simulink model "IdmEstimation_Cogen"  (R2017b)
settings: Solver=FixedStepDiscrete  StartTime=0.0  StopTime=SimTime  FixedStep=0.01  RelTol=1e-3
values from neighbouring files (symbols this model uses):
  BaseMap_CoastAccdiff_Index = (0:0.5:3.5)'    [IdmDev_MdlClassification.m]    (also in IdmParam.mat = [0 0.5 1 1.5 2 2.5 3 3.5]; IdmParam_Integ.mat = [0 0.5 1 1.5 2 2.5 3 3.5])
  BaseMap_CoastSpeed_Index = (5:5:40)'    [IdmDev_MdlClassification.m]    (also in IdmParam.mat = [5 10 15 20 25 30 35 40]; IdmParam_Integ.mat = [5 10 15 20 25 30 35 40])
  LrnConfig =     [ModelConfig.mat]
  ModelConfig =     [ModelConfig.mat]
  OnlineConfig =     [ModelConfig.mat]
  ParamCase = Fcn_ParamSelect(Param,Index_case)    [IdmDev_LearnSILsValidation.m]    (also in IdmDev_LearningOnlineSimulation.m)
undefined symbols (not defined in the file or in its folder): acc_veh, dis_veh, vel_veh
libraries: simulink x7
(part 2 of 2)

== system IdmEstimation_Cogen/IdmLrn_ParameterUpdate/Parameter update/MaxAccUpdate ==
  MaxAccRef : Inport
  MaxAcc : Inport  Port=2
  LrnFac : Inport  Port=3
  In4 : Inport  Port=4
  Constant1 : Constant  Value=LrnConfig.ExpUpdateGain
  Constant2 : Constant  Value=LrnConfig.LrnSwt
  Data Store Read : DataStoreRead  DataStoreName=IdmLrn_EcpParamVec_MaxAcc
  Data Store Write1 : DataStoreWrite  DataStoreName=IdmLrn_EcpParamVec_MaxAcc
  Divide : Product  Inputs=*/
  Product : Product
  Sum : Sum  Inputs=|+-
  Sum1 : Sum  Inputs=|++
  Switch : Switch  Criteria=u2 > Threshold  Threshold=0.5
  To Workspace : ToWorkspace  VariableName=LrnResult_EcpParamVec_MaxAcc  SaveFormat=Structure With Time  SampleTime=-1
  wires:
  Product/1 -> Divide/1  "TargetDelta"
  Sum/1 -> Product/1
  MaxAcc/1 -> Sum/2
  Switch/1 -> Product/2
  MaxAccRef/1 -> Sum/1
  LrnFac/1 -> Divide/2
  Divide/1 -> Sum1/1  "LrnValueVec"
  Data Store Read/1 -> Sum1/2
  Sum1/1 -> To Workspace/1, Data Store Write1/1
  Constant2/1 -> Switch/2
  In4/1 -> Switch/3
  Constant1/1 -> Switch/1

== system IdmEstimation_Cogen/IdmLrn_ParameterUpdate/Parameter update/TpDeltaUpdate ==
  TpStallRef : Inport
  TpStall : Inport  Port=2
  LrnFac : Inport  Port=3
  In4 : Inport  Port=4
  Constant : Constant  Value=LrnConfig.ExpUpdateGain
  Constant1 : Constant  Value=LrnConfig.LrnSwt
  Data Store Read2 : DataStoreRead  DataStoreName=IdmLrn_EcpParamVec_TpDelta
  Data Store Write3 : DataStoreWrite  DataStoreName=IdmLrn_EcpParamVec_TpDelta
  Divide : Product  Inputs=*/
  Product : Product
  Sum : Sum  Inputs=|+-
  Sum1 : Sum  Inputs=|++
  Switch : Switch  Criteria=u2 > Threshold  Threshold=0.5
  To Workspace : ToWorkspace  VariableName=LrnResult_EcpParamVec_TpDelta  SaveFormat=Structure With Time  SampleTime=-1
  wires:
  Sum1/1 -> To Workspace/1, Data Store Write3/1
  Data Store Read2/1 -> Sum1/2
  Divide/1 -> Sum1/1  "LrnValueVec"
  LrnFac/1 -> Divide/2
  TpStallRef/1 -> Sum/1
  Switch/1 -> Product/2
  TpStall/1 -> Sum/2
  Sum/1 -> Product/1
  Product/1 -> Divide/1  "TargetDelta"
  Constant1/1 -> Switch/2
  In4/1 -> Switch/3
  Constant/1 -> Switch/1

== system IdmEstimation_Cogen/IdmLrn_ParameterUpdate/Parameter update/TpInitUpdate ==
  TpInitRef : Inport
  TpInit : Inport  Port=2
  LrnFac : Inport  Port=3
  In4 : Inport  Port=4
  Constant : Constant  Value=LrnConfig.ExpUpdateGain
  Constant1 : Constant  Value=LrnConfig.LrnSwt
  Data Store Read2 : DataStoreRead  DataStoreName=IdmLrn_EcpParamVec_TpInit
  Data Store Write2 : DataStoreWrite  DataStoreName=IdmLrn_EcpParamVec_TpInit
  Display : Display
  Divide : Product  Inputs=*/
  Product : Product
  Sum : Sum  Inputs=|+-
  Sum1 : Sum  Inputs=|++
  Switch : Switch  Criteria=u2 > Threshold  Threshold=0.5
  To Workspace : ToWorkspace  VariableName=LrnResult_EcpParamVec_TpInit  SaveFormat=Structure With Time  SampleTime=-1
  wires:
  Product/1 -> Divide/1  "TargetDelta"
  Sum/1 -> Display/1, Product/1
  TpInit/1 -> Sum/2
  Constant/1 -> Switch/1
  TpInitRef/1 -> Sum/1
  LrnFac/1 -> Divide/2
  Divide/1 -> Sum1/1  "LrnValueVec"
  Data Store Read2/1 -> Sum1/2
  Sum1/1 -> To Workspace/1, Data Store Write2/1
  Constant1/1 -> Switch/2
  In4/1 -> Switch/3
  Switch/1 -> Product/2

== system IdmEstimation_Cogen/IdmEst_AccEstimation/Model profile update/Model profile update - Coast state/DisAdjCalc ==
  Constant : Constant  Value=0
  Mod_DisAdj : Outport
  wires:
  Constant/1 -> Mod_DisAdj/1

== system IdmEstimation_Cogen/IdmEst_AccEstimation/Model profile update/Model profile update - Coast state/DisDelCalc ==
  Constant : Constant  Value=0
  Mod_DisDel : Outport
  wires:
  Constant/1 -> Mod_DisDel/1

== system IdmEstimation_Cogen/IdmEst_AccEstimation/Model profile update/Model profile update - Coast state/RefAccCalc ==
  note: tmpLoc_ModProf_acc_ref(index_curstep+1) = -0.5*tmpLoc_Mod_vel_est(index_curstep+1).^2/(tmpLoc_Mod_dis_est(index_curstep+1) - DrvConfig.StopDis);
  Mod_VelEstPri : Inport
  Mod_DisEstPri : Inport  Port=2
  Constant : Constant  Value=ModelConfig.StopDis
  Constant1 : Constant  Value=-0.5
  Product : Product
  Product1 : Product  Inputs=**/
  Sum : Sum  Inputs=|+-
  Mod_AccRef : Outport
  wires:
  Mod_VelEstPri/1 -> Product/2, Product/1
  Product/1 -> Product1/2
  Constant1/1 -> Product1/1
  Mod_DisEstPri/1 -> Sum/1
  Constant/1 -> Sum/2
  Sum/1 -> Product1/3
  Product1/1 -> Mod_AccRef/1

== system IdmEstimation_Cogen/IdmEst_AccEstimation/Model profile update/Model profile update - Coast state/RefVelCalc ==
  Mod_VelRefPri : Inport
  AccEst : Inport  Port=2
  Constant : Constant  Value=OnlineConfig.Ts
  Product : Product
  Sum : Sum  Inputs=|++
  Mod_VelRef : Outport
  wires:
  Mod_VelRefPri/1 -> Sum/1
  Product/1 -> Sum/2
  Sum/1 -> Mod_VelRef/1
  Constant/1 -> Product/2
  AccEst/1 -> Product/1

== system IdmEstimation_Cogen/IdmEst_AccEstimation/Model profile update/Model profile update - Disadj state/DisAdjCalc ==
  Mod_DisEstPri : Inport
  Mod_DisAdj : Outport
  wires:
  Mod_DisEstPri/1 -> Mod_DisAdj/1

== system IdmEstimation_Cogen/IdmEst_AccEstimation/Model profile update/Model profile update - Disadj state/DisDelCalc ==
  Mod_DisDelPri : Inport
  ModelParam : Inport  Port=2
  In3 : Inport  Port=3
  Product : Product
  Selector : Selector  InputPortWidth=OnlineConfig.CalcParamSize  IndexOptions=Index vector (dialog)  Indices=OnlineConfig.CalcParamIndex.AccdDisAdj  OutputSizes=1
  Sum : Sum  Inputs=|++
  Mod_DisDel : Outport
  wires:
  Sum/1 -> Mod_DisDel/1
  ModelParam/1 -> Selector/1
  Selector/1 -> Product/1  "ModelParam_AccDiff"
  Mod_DisDelPri/1 -> Sum/1
  In3/1 -> Product/2
  Product/1 -> Sum/2

== system IdmEstimation_Cogen/IdmEst_AccEstimation/Model profile update/Model profile update - Disadj state/RefAccCalc ==
  note: tmpLoc_ModProf_acc_ref(index_curstep+1) = -0.5*tmpLoc_Mod_vel_est(index_curstep+1).^2/(tmpLoc_Mod_dis_est(index_curstep+1) - DrvConfig.StopDis);
  Mod_VelEstPri : Inport
  Mod_DisEstPri : Inport  Port=2
  Constant : Constant  Value=ModelConfig.StopDis
  Constant1 : Constant  Value=-0.5
  Product : Product
  Product1 : Product  Inputs=**/
  Sum : Sum  Inputs=|+-
  Mod_AccRef : Outport
  wires:
  Mod_VelEstPri/1 -> Product/2, Product/1
  Product/1 -> Product1/2
  Constant1/1 -> Product1/1
  Mod_DisEstPri/1 -> Sum/1
  Constant/1 -> Sum/2
  Sum/1 -> Product1/3
  Product1/1 -> Mod_AccRef/1

== system IdmEstimation_Cogen/IdmEst_AccEstimation/Model profile update/Model profile update - Disadj state/RefVelCalc ==
  Mod_VelEstPri : Inport
  Mod_DisEstPri : Inport  Port=2
  Mod_DisAdjPri : Inport  Port=3
  ModParam : Inport  Port=4
  Constant1 : Constant  Value=1/ModelConfig.Delta
  Math Function : Math  Operator=pow  SaturateOnIntegerOverflow=on
  Math Function1 : Math  Operator=square  SaturateOnIntegerOverflow=on
  Product : Product  Inputs=*/
  Product1 : Product  Inputs=*/
  Saturation : Saturate  UpperLimit=inf  LowerLimit=0.00001
  Selector : Selector  InputPortWidth=OnlineConfig.CalcParamSize  IndexOptions=Index vector (dialog)  Indices=OnlineConfig.CalcParamIndex.AccrStall  OutputSizes=1
  Sum1 : Sum  Inputs=|+-
  Mod_VelRef : Outport
  wires:
  Product/1 -> Mod_VelRef/1
  Mod_VelEstPri/1 -> Product/1
  ModParam/1 -> Selector/1
  Selector/1 -> Sum1/1  "ModParam_AccRatioFacStall"
  Mod_DisAdjPri/1 -> Product1/1
  Mod_DisEstPri/1 -> Product1/2
  Sum1/1 -> Saturation/1
  Constant1/1 -> Math Function/2
  Math Function/1 -> Product/2
  Product1/1 -> Math Function1/1
  Math Function1/1 -> Sum1/2
  Saturation/1 -> Math Function/1

== system IdmEstimation_Cogen/IdmEst_AccEstimation/Model profile update/Model profile update - Initial state/DisAdjCalc ==
  Constant : Constant  Value=0
  Mod_DisAdj : Outport
  wires:
  Constant/1 -> Mod_DisAdj/1

== system IdmEstimation_Cogen/IdmEst_AccEstimation/Model profile update/Model profile update - Initial state/DisDelCalc ==
  Constant : Constant  Value=0
  Mod_DisDel : Outport
  wires:
  Constant/1 -> Mod_DisDel/1

== system IdmEstimation_Cogen/IdmEst_AccEstimation/Model profile update/Model profile update - Initial state/RefAccCalc ==
  note: tmpLoc_ModProf_acc_ref(index_curstep+1) = -0.5*tmpLoc_Mod_vel_est(index_curstep+1).^2/(tmpLoc_Mod_dis_est(index_curstep+1) - DrvConfig.StopDis);
  Mod_VelEstPri : Inport
  Mod_DisEstPri : Inport  Port=2
  Constant : Constant  Value=ModelConfig.StopDis
  Constant1 : Constant  Value=-0.5
  Product : Product
  Product1 : Product  Inputs=**/
  Sum : Sum  Inputs=|+-
  Mod_AccRef : Outport
  wires:
  Mod_VelEstPri/1 -> Product/2, Product/1
  Product/1 -> Product1/2
  Constant1/1 -> Product1/1
  Mod_DisEstPri/1 -> Sum/1
  Constant/1 -> Sum/2
  Sum/1 -> Product1/3
  Product1/1 -> Mod_AccRef/1

== system IdmEstimation_Cogen/IdmEst_AccEstimation/Model profile update/Model profile update - Initial state/RefVelCalc ==
  Mod_VelEstPri : Inport
  ModelParam : Inport  Port=2
  Divide : Product  Inputs=*/
  Selector : Selector  InputPortWidth=OnlineConfig.CalcParamSize  IndexOptions=Index vector (dialog)  Indices=OnlineConfig.CalcParamIndex.VelRatio  OutputSizes=1
  Mod_VelRef : Outport
  wires:
  Divide/1 -> Mod_VelRef/1
  Selector/1 -> Divide/2
  Mod_VelEstPri/1 -> Divide/1
  ModelParam/1 -> Selector/1

== system IdmEstimation_Cogen/IdmEst_AccEstimation/Model profile update/Model profile update - Term state/DisAdjCalc ==
  Mod_DisEstPri : Inport
  Mod_DisAdj : Outport
  wires:
  Mod_DisEstPri/1 -> Mod_DisAdj/1

== system IdmEstimation_Cogen/IdmEst_AccEstimation/Model profile update/Model profile update - Term state/DisDelCalc ==
  AccEst : Inport
  AccRef : Inport  Port=2
  Mod_DisDelPri : Inport  Port=3
  Constant : Constant  Value=ModelConfig.AdjDisGainTerm
  Product : Product
  Sum1 : Sum  Inputs=|++
  Sum2 : Sum  Inputs=|+-
  Mod_DisDel : Outport
  wires:
  Sum1/1 -> Mod_DisDel/1
  Constant/1 -> Product/2
  Product/1 -> Sum1/2
  Mod_DisDelPri/1 -> Sum1/1
  AccEst/1 -> Sum2/1
  AccRef/1 -> Sum2/2
  Sum2/1 -> Product/1

== system IdmEstimation_Cogen/IdmEst_AccEstimation/Model profile update/Model profile update - Term state/RefAccCalc ==
  note: tmpLoc_ModProf_acc_ref(index_curstep+1) = -0.5*tmpLoc_Mod_vel_est(index_curstep+1).^2/(tmpLoc_Mod_dis_est(index_curstep+1) - DrvConfig.StopDis);
  Mod_VelEstPri : Inport
  Mod_DisEstPri : Inport  Port=2
  Constant : Constant  Value=ModelConfig.StopDis
  Constant1 : Constant  Value=-0.5
  Product : Product
  Product1 : Product  Inputs=**/
  Sum : Sum  Inputs=|+-
  Mod_AccRef : Outport
  wires:
  Mod_VelEstPri/1 -> Product/2, Product/1
  Product/1 -> Product1/2
  Constant1/1 -> Product1/1
  Mod_DisEstPri/1 -> Sum/1
  Constant/1 -> Sum/2
  Sum/1 -> Product1/3
  Product1/1 -> Mod_AccRef/1

== system IdmEstimation_Cogen/IdmEst_AccEstimation/Model profile update/Model profile update - Term state/RefVelCalc ==
  Mod_VelEstPri : Inport
  Mod_DisEstPri : Inport  Port=2
  Mod_DisAdjPri : Inport  Port=3
  ModParam : Inport  Port=4
  Constant : Constant  Value=1/ModelConfig.Delta
  Math Function : Math  Operator=pow  SaturateOnIntegerOverflow=on
  Math Function1 : Math  Operator=square  SaturateOnIntegerOverflow=on
  Product : Product  Inputs=*/
  Product1 : Product  Inputs=*/
  Saturation : Saturate  UpperLimit=inf  LowerLimit=0.00001
  Selector : Selector  InputPortWidth=OnlineConfig.CalcParamSize  IndexOptions=Index vector (dialog)  Indices=OnlineConfig.CalcParamIndex.AccrStall  OutputSizes=1
  Sum1 : Sum  Inputs=|+-
  Mod_VelRef : Outport
  wires:
  Product/1 -> Mod_VelRef/1
  Mod_VelEstPri/1 -> Product/1
  ModParam/1 -> Selector/1
  Selector/1 -> Sum1/1  "ModParam_AccRatioFacStall"
  Mod_DisAdjPri/1 -> Product1/1
  Mod_DisEstPri/1 -> Product1/2
  Sum1/1 -> Saturation/1
  Constant/1 -> Math Function/2
  Math Function/1 -> Product/2
  Product1/1 -> Math Function1/1
  Math Function1/1 -> Sum1/2
  Saturation/1 -> Math Function/1

== system IdmEstimation_Cogen/IdmEst_AccEstimation/Model profile update/Model profile update - Veladj state/DisAdjCalc ==
  Mod_DisEstPri : Inport
  ModParam : Inport  Port=2
  Constant : Constant  Value=ModelConfig.VelAdjFac
  Product : Product  Inputs=**/
  Selector : Selector  InputPortWidth=OnlineConfig.CalcParamSize  IndexOptions=Index vector (dialog)  Indices=OnlineConfig.CalcParamIndex.DisStall  OutputSizes=1
  Selector1 : Selector  InputPortWidth=OnlineConfig.CalcParamSize  IndexOptions=Index vector (dialog)  Indices=OnlineConfig.CalcParamIndex.VelStall  OutputSizes=1
  Sum : Sum  Inputs=|+-
  Mod_DisAdj : Outport
  wires:
  ModParam/1 -> Selector1/1, Selector/1
  Selector/1 -> Sum/1  "ModParam_DisStall"
  Selector1/1 -> Product/2  "ModParam_VelStall"
  Mod_DisEstPri/1 -> Sum/2
  Sum/1 -> Product/1
  Constant/1 -> Product/3
  Product/1 -> Mod_DisAdj/1

== system IdmEstimation_Cogen/IdmEst_AccEstimation/Model profile update/Model profile update - Veladj state/DisDelCalc ==
  Constant : Constant  Value=0
  Mod_DisDel : Outport
  wires:
  Constant/1 -> Mod_DisDel/1

== system IdmEstimation_Cogen/IdmEst_AccEstimation/Model profile update/Model profile update - Veladj state/RefAccCalc ==
  note: tmpLoc_ModProf_acc_ref(index_curstep+1) = -0.5*tmpLoc_Mod_vel_est(index_curstep+1).^2/(tmpLoc_Mod_dis_est(index_curstep+1) - DrvConfig.StopDis);
  Mod_VelEstPri : Inport
  Mod_DisEstPri : Inport  Port=2
  Constant : Constant  Value=ModelConfig.StopDis
  Constant1 : Constant  Value=-0.5
  Product : Product
  Product1 : Product  Inputs=**/
  Sum : Sum  Inputs=|+-
  Mod_AccRef : Outport
  wires:
  Mod_VelEstPri/1 -> Product/2, Product/1
  Product/1 -> Product1/2
  Constant1/1 -> Product1/1
  Mod_DisEstPri/1 -> Sum/1
  Constant/1 -> Sum/2
  Sum/1 -> Product1/3
  Product1/1 -> Mod_AccRef/1

== system IdmEstimation_Cogen/IdmEst_AccEstimation/Model profile update/Model profile update - Veladj state/RefVelCalc ==
  Mod_VelEstPri : Inport
  Mod_DisEstPri : Inport  Port=2
  Mod_DisAdjPri : Inport  Port=3
  ModParam : Inport  Port=4
  Constant : Constant  Value=1/ModelConfig.Delta
  Math Function : Math  Operator=pow  SaturateOnIntegerOverflow=on
  Math Function1 : Math  Operator=square  SaturateOnIntegerOverflow=on
  Product : Product  Inputs=*/
  Product1 : Product  Inputs=*/
  Saturation : Saturate  UpperLimit=inf  LowerLimit=0.00001
  Selector : Selector  InputPortWidth=OnlineConfig.CalcParamSize  IndexOptions=Index vector (dialog)  Indices=OnlineConfig.CalcParamIndex.AccrStall  OutputSizes=1
  Sum1 : Sum  Inputs=|+-
  Mod_VelRef : Outport
  wires:
  Product/1 -> Mod_VelRef/1
  Mod_VelEstPri/1 -> Product/1
  ModParam/1 -> Selector/1
  Selector/1 -> Sum1/1  "ModParam_AccRatioFacStall"
  Mod_DisAdjPri/1 -> Product1/1
  Mod_DisEstPri/1 -> Product1/2
  Sum1/1 -> Saturation/1
  Constant/1 -> Math Function/2
  Math Function/1 -> Product/2
  Product1/1 -> Math Function1/1
  Math Function1/1 -> Sum1/2
  Saturation/1 -> Math Function/1

== system IdmEstimation_Cogen/IdmEst_AccEstimation/Parameter management/DisAdjStateOn/If Action Subsystem2 ==
  In1 : Inport
  Action Port : ActionPort  ActionType=else
  Out1 : Outport
  wires:
  In1/1 -> Out1/1

== system IdmEstimation_Cogen/IdmEst_AccEstimation/Parameter management/DisAdjStateOn/If Action Subsystem3 ==
  ModelProPri : Inport
  Action Port : ActionPort  ActionType=then
  Demux : Demux  Outputs=2
  Sum2 : Sum  Inputs=|+-
  ModelParam_DisAdjInit : Outport
  wires:
  Demux/1 -> Sum2/1  "acc_est"
  ModelProPri/1 -> Demux/1
  Demux/2 -> Sum2/2  "acc_ref"
  Sum2/1 -> ModelParam_DisAdjInit/1

== system IdmEstimation_Cogen/IdmEst_AccEstimation/Parameter management/InitStateOn/If Action Subsystem4 ==
  ModelParamCalc_Pri : Inport
  MaxAcc : Inport  Port=2
  In3 : Inport  Port=3
  Action Port : ActionPort  ActionType=else
  Constant : Constant  Value=1/ModelConfig.Delta
  Constant1 : Constant  Value=ModelConfig.Delta
  Demux : Demux  Outputs=2
  Math Function2 : Math  Operator=pow  SaturateOnIntegerOverflow=on
  Math Function3 : Math  Operator=pow  SaturateOnIntegerOverflow=on
  Mux : Mux  Inputs=2
  Product2 : Product  Inputs=*/
  Sum : Sum  Inputs=|+-
  Out1 : Outport
  Out2 : Outport  Port=2
  wires:
  ModelParamCalc_Pri/1 -> Demux/1
  Demux/1 -> Math Function2/1  "VelRatio_Pri"
  Demux/2 -> Mux/2, Product2/1  "AccDel"
  Mux/1 -> Out1/1
  Constant1/1 -> Math Function2/2
  Math Function2/1 -> Sum/1
  Product2/1 -> Sum/2
  Sum/1 -> Math Function3/1
  Constant/1 -> Math Function3/2
  Math Function3/1 -> Mux/1
  MaxAcc/1 -> Product2/2
  In3/1 -> Out2/1

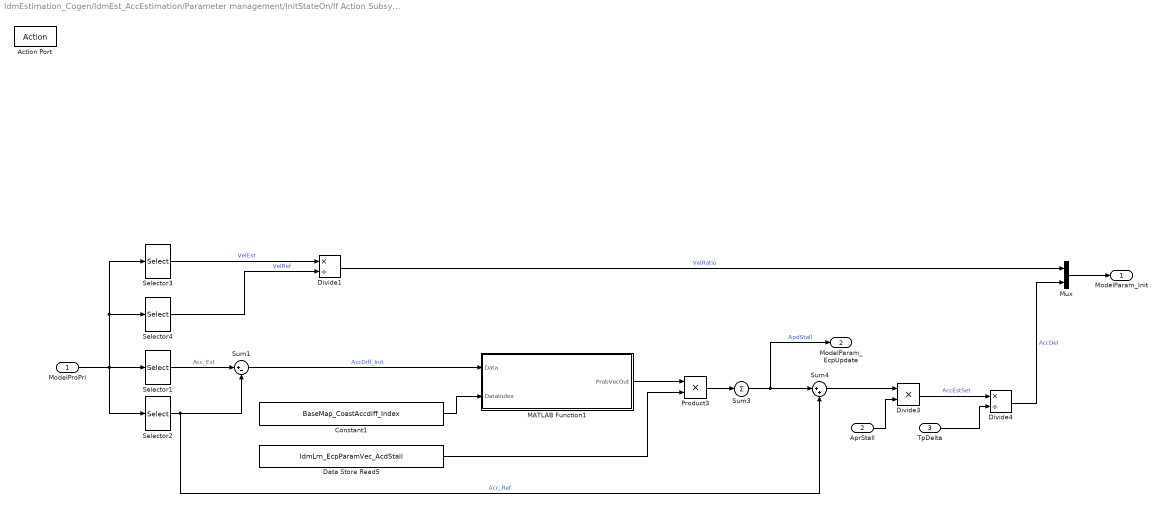
== system IdmEstimation_Cogen/IdmEst_AccEstimation/Parameter management/InitStateOn/If Action Subsystem5 ==
  ModelProPri : Inport
  AprStall : Inport  Port=2
  TpDelta : Inport  Port=3
  Action Port : ActionPort  ActionType=then
  Constant1 : Constant  Value=BaseMap_CoastAccdiff_Index
  Data Store Read5 : DataStoreRead  DataStoreName=IdmLrn_EcpParamVec_AcdStall
  Divide1 : Product  Inputs=*/
  Divide3 : Product
  Divide4 : Product  Inputs=*/
  MATLAB Function1 : MATLAB Function  TreatAsAtomicUnit=on
  Mux : Mux  Inputs=2
  Product3 : Product
  Selector1 : Selector  InputPortWidth=7  IndexOptions=Index vector (dialog)  Indices=1  OutputSizes=1
  Selector2 : Selector  InputPortWidth=7  IndexOptions=Index vector (dialog)  Indices=2  OutputSizes=1
  Selector3 : Selector  InputPortWidth=7  IndexOptions=Index vector (dialog)  Indices=3  OutputSizes=1
  Selector4 : Selector  InputPortWidth=7  IndexOptions=Index vector (dialog)  Indices=4  OutputSizes=1
  Sum1 : Sum  Inputs=|+-
  Sum3 : Sum  Inputs=1
  Sum4 : Sum  Inputs=|++
  ModelParam_Init : Outport
  ModelParam_EcpUpdate : Outport  Port=2
  wires:
  ModelProPri/1 -> Selector3/1, Selector4/1, Selector2/1, Selector1/1
  Mux/1 -> ModelParam_Init/1
  Divide4/1 -> Mux/2  "AccDel"
  Divide1/1 -> Mux/1  "VelRatio"
  Constant1/1 -> MATLAB Function1/2(DataIndex)
  Selector1/1 -> Sum1/1  "Acc_Est"
  Selector2/1 -> Sum4/2, Sum1/2  "Acc_Ref"
  Sum1/1 -> MATLAB Function1/1(Data)  "AccDiff_Init"
  Data Store Read5/1 -> Product3/2
  MATLAB Function1/1(ProbVecOut) -> Product3/1
  Product3/1 -> Sum3/1
  Sum3/1 -> ModelParam_EcpUpdate/1, Sum4/1  "ApdStall"
  Sum4/1 -> Divide3/1
  AprStall/1 -> Divide3/2
  Divide3/1 -> Divide4/1  "AccEstSet"
  TpDelta/1 -> Divide4/2
  Selector3/1 -> Divide1/1  "VelEst"
  Selector4/1 -> Divide1/2  "VelRef"

== system IdmEstimation_Cogen/IdmEst_AccEstimation/Parameter management/VelAdjStateOn/If Action Subsystem ==
  ModelProPri : Inport
  MaxAcc : Inport  Port=2
  Action Port : ActionPort  ActionType=then
  Constant2 : Constant
  Demux : Demux  Outputs=3
  Mux : Mux  Inputs=3
  Product : Product  Inputs=*/
  Saturation : Saturate  UpperLimit=inf  LowerLimit=0
  Sum1 : Sum  Inputs=|+-
  ModelParam_VelAdjInit : Outport
  wires:
  ModelProPri/1 -> Demux/1
  Demux/1 -> Product/1  "acc_est"
  Demux/2 -> Mux/2  "vel_est"
  Demux/3 -> Mux/3  "dis_est"
  MaxAcc/1 -> Product/2
  Product/1 -> Sum1/2
  Constant2/1 -> Sum1/1
  Sum1/1 -> Saturation/1
  Saturation/1 -> Mux/1  "AccRatioFactor_Stall"
  Mux/1 -> ModelParam_VelAdjInit/1

== system IdmEstimation_Cogen/IdmEst_AccEstimation/Parameter management/VelAdjStateOn/If Action Subsystem1 ==
  In1 : Inport
  Action Port : ActionPort  ActionType=else
  Out1 : Outport
  wires:
  In1/1 -> Out1/1

== stateflow chart IdmEstimation_Cogen/IdmMng_CoastingConditionManager/Chart ==
  state CoastInitState
    entry: stDrvState = 3;
    Local_InitTime = 1;
    during: stDrvState =3;
    Local_InitTime = Local_InitTime +1;
    exit: Local_InitTime = 0;
  state CoastState
    entry: stDrvState = OnlineConfig.DriveState.Braking;
    stCoastFlag = OnlineConfig.CoastFlag.Start;
    during: stDrvState = OnlineConfig.DriveState.Braking;
    stCoastFlag  = OnlineConfig.CoastFlag.None;
  state NormalState
    entry: stDrvState = OnlineConfig.DriveState.Driving;
    during: stDrvState = OnlineConfig.DriveState.Driving;
  state StopState
    entry: stDrvState = OnlineConfig.DriveState.Stop;
    stCoastFlag = OnlineConfig.CoastFlag.Stop;
    Local_StopTime = 1;
    during: stDrvState = OnlineConfig.DriveState.Stop;
    stCoastFlag = OnlineConfig.CoastFlag.None;
    Local_StopTime = Local_StopTime +1;
    exit: Local_StopTime = 0;
  NormalState -> CoastInitState : [[(Vel >= OnlineConfig.CoastCond.Vel)&& ...
      | (Aps <= OnlineConfig.CoastCond.Gas )] ]
  CoastInitState -> (junction 22) : [Local_InitTime >= OnlineConfig.CoastInitBuff]
  (default) -> NormalState
  (junction 22) -> NormalState [order 2]
  (junction 22) -> CoastState [order 1] : [Aps <= OnlineConfig.CoastCond.Gas ]
  CoastState -> NormalState [order 2] : [[Aps > OnlineConfig.CoastCond.Gas ] ]
  StopState -> NormalState : [(Local_StopTime >= OnlineConfig.StopCond.Time ) ...
      | &&(Vel >= OnlineConfig.StartCond.Vel)]
  CoastState -> StopState [order 1] : [(Dis <= OnlineConfig.StopCond.Dis+0.01)|| ...
      | (Vel <= OnlineConfig.StopCond.Vel+0.001)]
  data: Aps input; Vel input; Local_StopTime local; Dis input; OnlineConfig parameter; stDrvState output; stCoastFlag output; Local_InitTime local

== matlab function IdmEstimation_Cogen/IdmLrn_ParameterUpdate/End state/MATLAB Function ==
  data: BrakingDataArry input; Tp_Shift input; LrnParamVec output [1..6]; OnlineConfig parameter; LrnConfig parameter; TpDisAdj input; ModelConfig parameter; LrnProfAccFilt output; LrnProfAccRefFiltCompOut output; LrnProfAccRefFiltOut output
function [LrnParamVec,LrnProfAccFilt,LrnProfAccRefFiltCompOut,LrnProfAccRefFiltOut]= LrnParamCalc(BrakingDataArry, Tp_Shift, OnlineConfig, LrnConfig, TpDisAdj, ModelConfig)

persistent LrnProfVelRef;
persistent LrnProfVelDiffFilt;
persistent LrnProfAccRefFilt;
persistent LrnProfAccRefFiltComp;

if isempty(LrnProfVelRef)
    LrnProfVelRef = zeros(OnlineConfig.CoastingIndexSize,1);
end

if isempty(LrnProfAccRefFilt)
    LrnProfAccRefFilt = zeros(OnlineConfig.CoastingIndexSize,1);
end

if isempty(LrnProfVelDiffFilt)
    LrnProfVelDiffFilt = zeros(OnlineConfig.CoastingIndexSize,1);
end

if isempty(LrnProfAccRefFiltComp)
    LrnProfAccRefFiltComp = zeros(OnlineConfig.CoastingIndexSize,1);
end  

tmpBrk = Tp_Shift;
tmpFiltNum = LrnConfig.AccFiltNum;

VehData_acc = BrakingDataArry(:,1);
VehData_vel = BrakingDataArry(:,2);
VehData_dis = BrakingDataArry(:,3);
VehData_time = (OnlineConfig.Ts:OnlineConfig.Ts:OnlineConfig.CoastingIndexSize*OnlineConfig.Ts)';

LrnProfAccFilt = zeros(OnlineConfig.CoastingIndexSize,1);
for i = (tmpFiltNum+1):OnlineConfig.CoastingIndexSize-tmpFiltNum
    LrnProfAccFilt(i) = mean(VehData_acc(i-tmpFiltNum:i+tmpFiltNum));   
end

Lrn_ExpParam_MinAcc = min(LrnProfAccFilt);
Lrn_ExpParam_MaxAcc = -Lrn_ExpParam_MinAcc;

tmpVelEff = (1 - VehData_acc./Lrn_ExpParam_MaxAcc);
tmpVelEff(tmpVelEff<LrnConfig.VelEffMin) = LrnConfig.VelEffMin;
   
tmpTpStop = min(find((VehData_vel<LrnConfig.VelTerm) & (VehData_time>LrnConfig.CoastTime),1));

if isempty(tmpTpStop)
    [tmpDummy tmpTpStop] = min(VehData_vel);
end

% Reference velocity calculation
LrnProfVelRef = VehData_vel./(tmpVelEff).^(1/ModelConfig.Delta);        
LrnProfVelDiff = VehData_vel - LrnProfVelRef;

for i = (tmpFiltNum+1):OnlineConfig.CoastingIndexSize-tmpFiltNum
    LrnProfVelDiffFilt(i) = mean(LrnProfVelDiff(i-tmpFiltNum:i+tmpFiltNum));   
end
LrnProfAccRef = -0.5*VehData_vel.^2./(VehData_dis - ModelConfig.StopDis);

for i = (tmpFiltNum+1):OnlineConfig.CoastingIndexSize-tmpFiltNum
    LrnProfAccRefFilt(i) = mean(LrnProfAccRef(i-tmpFiltNum:i+tmpFiltNum));   
end

% Init point, Adjustment point calculation
% tmpTpInit = min(find(LrnProfVelDiffFilt(tmpFiltNum + 1:tmpTpStop)>=LrnProfVelDiffFilt( tmpFiltNum + 1)*LrnConfig.VelDifRatFac_Init,1));
% tmpTpInit = tmpFiltNum + tmpTpInit;
tmpTpInit = tmpBrk;
[tmpDummy tmpTpMax] = max(LrnProfVelDiffFilt(tmpTpInit:end));        
tmpTpDelta = tmpTpMax-1;
tmpTpStall = tmpTpInit+tmpTpMax-1;   
tmpTpAdj = TpDisAdj;
if (tmpTpAdj == 0)
    tmpTpAdj = tmpTpStall;
end

% Ref acc calculation
tmpLrnProfVelComp = cumtrapz(LrnProfAccFilt)*OnlineConfig.Ts;
[tmpDummy tmpStopPoint] = min(tmpLrnProfVelComp);
LrnProfVelComp = tmpLrnProfVelComp - tmpDummy;
tmpLrnProfDisComp = cumtrapz(LrnProfVelComp)*0.01;
LrnProfDisComp = tmpLrnProfDisComp(tmpStopPoint) - tmpLrnProfDisComp;
LrnProfAccRefFiltComp = -0.5*LrnProfVelComp.^2./LrnProfDisComp;
LrnProfAccRefFiltComp(tmpTpStop:end) = LrnProfAccRefFiltComp(tmpTpStop);
% Term point ref
tmpAccCompPtSt = min(tmpTpAdj,tmpTpStall) + LrnConfig.TermBuff;
tmpTpAdjRefIndex = find(abs(LrnProfAccRefFiltComp(tmpAccCompPtSt:tmpTpStop) - LrnProfAccFilt(tmpAccCompPtSt:tmpTpStop))<=LrnConfig.AdjAccDiff , 1);
if isempty(tmpTpAdjRefIndex)
    tmpTpAdjRefIndex = tmpTpStop;
end
tmpTpAdjRef = min(tmpTpAdjRefIndex);
tmpTpTermRef = tmpAccCompPtSt+tmpTpAdjRef-1;

% Accr
tmpAppStall = mean(LrnProfAccFilt(tmpTpStall-LrnConfig.AcrCalcWindow:tmpTpStall+LrnConfig.AcrCalcWindow));
tmpAppRefStall = LrnProfAccRefFiltComp(tmpTpStall);
tmpAppRefInit = LrnProfAccRefFiltComp(tmpTpInit);

Lrn_ExpParam_TpInit = tmpTpInit;
Lrn_ExpParam_TpDelta = tmpTpDelta;
Lrn_ExpParam_VpStall = LrnProfVelRef(tmpTpStall);
Lrn_ExpParam_AprStall = tmpAppStall/tmpAppRefStall;
Lrn_ExpParam_TpTermRef = tmpTpTermRef;
Lrn_ExpParam_ApdStall = tmpAppRefStall - tmpAppRefInit;

LrnParamVec  = [Lrn_ExpParam_TpInit Lrn_ExpParam_TpDelta Lrn_ExpParam_ApdStall Lrn_ExpParam_AprStall Lrn_ExpParam_MaxAcc Lrn_ExpParam_TpTermRef];
    
LrnProfAccRefFiltCompOut = LrnProfAccRefFiltComp;    
LrnProfAccRefFiltOut = LrnProfVelDiffFilt;

== stateflow chart IdmEstimation_Cogen/IdmEst_AccEstimation/State definition/Chart ==
  state StateChart
    state StateDefinition [parallel]
      settings: executionOrder=2
      state CoastState
        entry: stState = ModelConfig.stState.Coast;
        stStateFlag = ModelConfig.stStateFlag.Coast;
        during: stStateFlag = 0;
      state InitialState
        entry: stState = ModelConfig.stState.Init;
        stStateFlag = ModelConfig.stStateFlag.Init;
        during: stStateFlag = 0;
      state VelAdjState
        entry: stState = ModelConfig.stState.Veladj;
        stStateFlag = ModelConfig.stStateFlag.VeladjInit;
        during: stStateFlag = 0;
      state DisAdjState_OverCase
        entry: stState = ModelConfig.stState.Disadj;
        stStateFlag = ModelConfig.stStateFlag.DisadjInit;
        during: stStateFlag = 0;
      state DisAdjState_UnderCase
        entry: stState = ModelConfig.stState.Disadj;
        stStateFlag = ModelConfig.stStateFlag.DisadjInit;
        during: stStateFlag = 0;
      state TermState
        entry: stState = ModelConfig.stState.Term;
        stStateFlag = ModelConfig.stStateFlag.TermInit;
        during: stStateFlag = 0;
      state EndState
        entry: stState = ModelConfig.stState.End;
        stStateFlag = ModelConfig.stStateFlag.End;
        during: stStateFlag = 0;
      (default) -> CoastState
      CoastState -> EndState [order 2] : [DrvStateFlag == OnlineConfig.CoastFlag.Stop]
      EndState -> CoastState : [DrvStateFlag ==OnlineConfig.CoastFlag.Start]
      TermState -> CoastState [order 2] : [DrvStateFlag ==OnlineConfig.CoastFlag.Start]
      DisAdjState_OverCase -> CoastState [order 2] : [DrvStateFlag ==OnlineConfig.CoastFlag.Start]
      CoastState -> InitialState [order 1] : [((IndexTimeStep >= Param_Tp_Init)&&(IndexTimeStep > 0))]
      VelAdjState -> CoastState [order 2] : [DrvStateFlag ==OnlineConfig.CoastFlag.Start]
      DisAdjState_UnderCase -> CoastState [order 2] : [DrvStateFlag ==OnlineConfig.CoastFlag.Start]
      InitialState -> VelAdjState : [([LocParam_AccInitRef>LocParam_AccEst])||(IndexTimeStep > Param_Tp_Init + Param_Tp_Delta + ModelConfig.InitBuffTime)]
      VelAdjState -> (junction 51) [order 1] : [LocParam_DisEst<=LocParam_DisAdj]
      (junction 51) -> DisAdjState_UnderCase [order 1] : [LocParam_AccEst<=LocParam_AccRef]
      (junction 51) -> DisAdjState_OverCase [order 2]
      DisAdjState_OverCase -> EndState [order 3] : [(DrivingState ==OnlineConfig.DriveState.Driving)||(DrvStateFlag ==OnlineConfig.CoastFlag.Stop)]
      DisAdjState_OverCase -> TermState [order 1] : [LocParam_AccEst<=LocParam_AccRef]
      DisAdjState_UnderCase -> TermState [order 1] : [LocParam_AccEst>=LocParam_AccRef]
      DisAdjState_UnderCase -> EndState [order 3] : [(DrvStateFlag ==OnlineConfig.CoastFlag.Stop)||(DrivingState ==OnlineConfig.DriveState.Driving)]
      TermState -> EndState [order 1] : [(LocParam_VelEst<= 0.1)||(LocParam_DisEst<=0.5)]
    state DataArrangeState [parallel]
      settings: executionOrder=1
      state StateDataArrange
        during:
        LocParam_AccEst = ModelProfile(1);
        LocParam_AccRef = ModelProfile(2);
        LocParam_VelEst = ModelProfile(3);
        LocParam_DisEst = ModelProfile(5);
        LocParam_DisAdj = ModelProfile(6);
        LocParam_AccInitRef  = LocParam_AccRef * Param_Acr_Stall;
      (default) -> StateDataArrange
  data: DrvStateFlag input; DrivingState input; stState output; IndexTimeStep input; ModelProfile input; LocParam_AccEst local; LocParam_AccRef local; LocParam_DisAdj local; LocParam_DisEst local; LocParam_AccInitRef local; ModelConfig parameter; stStateFlag output; Param_Tp_Init input; Param_Tp_Delta input; Param_Acr_Stall input; LocParam_VelEst local; OnlineConfig parameter

== matlab function IdmEstimation_Cogen/IdmLrn_ParameterUpdate/Parameter update/MATLAB Function ==
  data: ProbVec input; LrnParamFacOut output; LrnConfig parameter
function LrnParamFacOut = ProbDecoding(ProbVec,LrnConfig)

persistent LrnParamFac;
if isempty(LrnParamFac)
    LrnParamFac = zeros(8,1);
end

persistent ProbSumEx;
if isempty(ProbSumEx)
    ProbSumEx = zeros(8,1);
end

IndexSet = 1:LrnConfig.DataIndexLength;

for i=1:LrnConfig.DataIndexLength
    ProbSumEx(i) = sum( ProbVec(IndexSet ~= i) );    
end

TmpParamSum = sum(ProbVec./ProbSumEx);

for i=1:LrnConfig.DataIndexLength
    LrnParamFac(i) = ProbSumEx(i)*TmpParamSum;
end    

LrnParamFacOut = LrnParamFac;

== matlab function IdmEstimation_Cogen/BrakingDataStorage/Start state/MATLAB Function ==
  data: veh_state input; BrakingDataOut output; OnlineConfig parameter
function BrakingDataOut = DataArrangement(veh_state, OnlineConfig)

persistent DataArry;
persistent step_index;

if isempty(DataArry)
    DataArry = zeros(OnlineConfig.CoastingIndexSize,3);
end

if isempty(step_index)
    step_index = 1;
end

DataArry(step_index,:) = veh_state(3:5);
BrakingDataOut = DataArry;

step_index = step_index+1;

end

== matlab function IdmEstimation_Cogen/IdmEst_CoastingStart/Explicit parameter selection/MATLAB Function1 ==
  data: Data input; DataIndex input; ProbVecOut output; LrnConfig parameter
function ProbVecOut = Fcn_FzProbBlending(Data,DataIndex,LrnConfig)
%FCN_BLENDING Summary of this function goes here
%   Detailed explanation goes here

persistent ProbVec
if isempty(ProbVec)
    ProbVec = zeros(LrnConfig.DataIndexLength,1);
end
IndexLength = LrnConfig.DataIndexLength;
Std = LrnConfig.ProbVecStdAcc;

% CoastSpeed = 0:0.01:100;

for i=1:IndexLength
    ProbVec(i) = 1/(Std*sqrt(2*pi))*exp(-0.5*((Data - DataIndex(i))./Std).^2);
end

ProbSum = sum(ProbVec);
ProbNorm = ProbVec./ProbSum;

ProbVecOut = ProbNorm;
end

== matlab function IdmEstimation_Cogen/IdmEst_CoastingStart/Explicit parameter selection/MATLAB Function ==
  data: Data input; DataIndex input; ProbVecOut output; LrnConfig parameter
function ProbVecOut = Fcn_FzProbBlending(Data,DataIndex,LrnConfig)
%FCN_BLENDING Summary of this function goes here
%   Detailed explanation goes here

persistent ProbVec
if isempty(ProbVec)
    ProbVec = zeros(LrnConfig.DataIndexLength,1);
end
IndexLength = LrnConfig.DataIndexLength;
Std = LrnConfig.ProbVecStdVel;

% CoastSpeed = 0:0.01:100;

for i=1:IndexLength
    ProbVec(i) = 1/(Std*sqrt(2*pi))*exp(-0.5*((Data - DataIndex(i))./Std).^2);
end

ProbSum = sum(ProbVec);
ProbNorm = ProbVec./ProbSum;

ProbVecOut = ProbNorm;
end

== matlab function IdmEstimation_Cogen/IdmLrn_ParameterUpdate/Parameter update/MATLAB Function1 ==
  data: ProbVec input; LrnParamFacOut output; LrnConfig parameter
function LrnParamFacOut = ProbDecoding(ProbVec,LrnConfig)

persistent LrnParamFac;
if isempty(LrnParamFac)
    LrnParamFac = zeros(8,1);
end

persistent ProbSumEx;
if isempty(ProbSumEx)
    ProbSumEx = zeros(8,1);
end

IndexSet = 1:LrnConfig.DataIndexLength;

for i=1:LrnConfig.DataIndexLength
    ProbSumEx(i) = sum( ProbVec(IndexSet ~= i) );    
end

TmpParamSum = sum(ProbVec./ProbSumEx);

for i=1:LrnConfig.DataIndexLength
    LrnParamFac(i) = ProbSumEx(i)*TmpParamSum;
end    

LrnParamFacOut = LrnParamFac;

== matlab function IdmEstimation_Cogen/IdmEst_AccEstimation/Parameter management/InitStateOn/If Action Subsystem5/MATLAB Function1 ==
  data: Data input; DataIndex input; ProbVecOut output; LrnConfig parameter
function ProbVecOut = Fcn_FzProbBlending(Data,DataIndex,LrnConfig)
%FCN_BLENDING Summary of this function goes here
%   Detailed explanation goes here

persistent ProbVec
if isempty(ProbVec)
    ProbVec = zeros(LrnConfig.DataIndexLength,1);
end
IndexLength = LrnConfig.DataIndexLength;
Std = LrnConfig.ProbVecStdAcc;

% CoastSpeed = 0:0.01:100;

for i=1:IndexLength
    ProbVec(i) = 1/(Std*sqrt(2*pi))*exp(-0.5*((Data - DataIndex(i))./Std).^2);
end

ProbSum = sum(ProbVec);
ProbNorm = ProbVec./ProbSum;

ProbVecOut = ProbNorm;
end

== matlab function IdmEstimation_Cogen/BrakingDataStorage/Start state/MATLAB Function1 ==
  data: Brk_Data input; Shift_TimeOut output
function Shift_TimeOut = fcn(Brk_Data)

persistent Shift_flag;
persistent step_index;
persistent Shift_Time;

if isempty(Shift_flag)
    Shift_flag = 0;
end

if isempty(Shift_Time)
    Shift_Time = 1;
end

if isempty(step_index)
    step_index = 1;
end


if (Brk_Data>2)&&(Shift_flag==0)
    Shift_Time = step_index;
    Shift_flag = 1;
end

Shift_TimeOut = Shift_Time;
step_index = step_index+1;


end

== matlab function IdmEstimation_Cogen/IdmEst_AccEstimation/Parameter management/MATLAB Function ==
  data: StateFlag input; PreStateArryOut output; StepIndex input
function PreStateArryOut = Fcn_PreStateDef(StateFlag,StepIndex)

persistent PreStateArry
if isempty(PreStateArry)
    PreStateArry = zeros(6,1);
end

if StateFlag == 1
    PreStateArry(1) = StepIndex;
elseif StateFlag == 2
    PreStateArry(2) = StepIndex;
elseif StateFlag == 3
    PreStateArry(3) = StepIndex;
elseif StateFlag == 4
    PreStateArry(4) = StepIndex;
elseif StateFlag == 5
    PreStateArry(5) = StepIndex;
elseif StateFlag == 6
    PreStateArry(6) = StepIndex;
end

PreStateArryOut = PreStateArry;
end
